simulink model "Sampling_Test"  (R2023b)
settings: Solver=VariableStepAuto  StartTime=0.0  StopTime=10.0  RelTol=1e-3
libraries: Pathfinding_lib x1
settings Model: Creator=FIRSTMentor  LastModifiedBy=FIRSTMentor

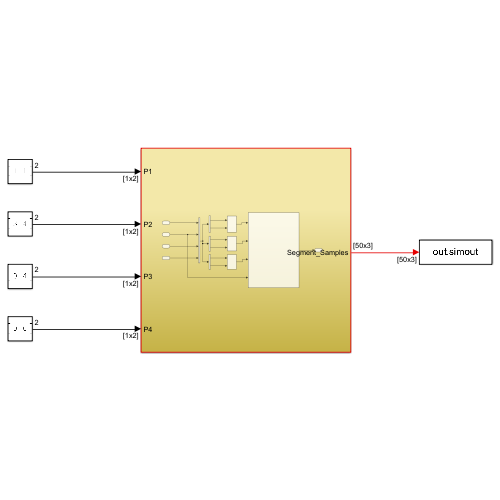
[thumbnail: Simulink's stored preview of the top-level diagram]
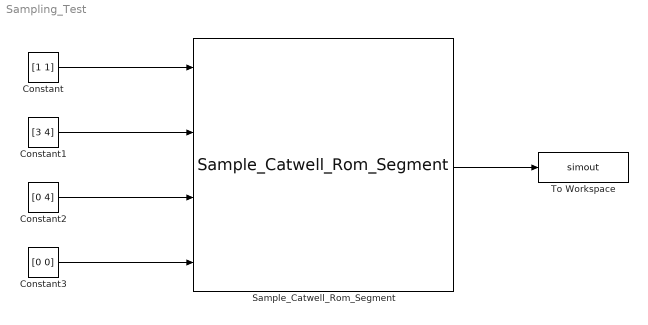
== system Sampling_Test ==
  Constant : Constant  Value=[1 1]
  Constant1 : Constant  Value=[3 4]
  Constant2 : Constant  Value=[0 4]
  Constant3 : Constant  Value=[0 0]
  Sample_Catwell_Rom_Segment : Pathfinding_lib/Sample_Catwell_Rom_Segment  SystemSampleTime=-1  VariantActivationTime=update diagram  AllowFlexibleInterface=on  Latency=0  AutoFrameSizeCalculation=off
  To Workspace : ToWorkspace  VariableName=simout  SampleTime=20
  wires:
  Constant/1 -> Sample_Catwell_Rom_Segment/1
  Constant1/1 -> Sample_Catwell_Rom_Segment/2
  Constant2/1 -> Sample_Catwell_Rom_Segment/3
  Constant3/1 -> Sample_Catwell_Rom_Segment/4
  Sample_Catwell_Rom_Segment/1 -> To Workspace/1
